simulink model "Child2"  (R2023a)
settings: Solver=FixedStepAuto  StartTime=0.0  StopTime=10.0  RelTol=1e-3
libraries: androidaudiovideolib x3, androidcommunicationlib x3, androidsensorlib x2, androiduilib x2, fuzblock x1
settings Model: Creator=srira  LastModifiedBy=srira
settings OptimizationCC: EnhancedBackFolding=on  PassReuseOutputArgsAs=Individual arguments  ZeroExternalMemoryAtStartup=off  ZeroInternalMemoryAtStartup=off  MaxStackSize=64  OptimizeBlockOrder=speed  DifferentSizesBufferReuse=on  OptimizationCustomize=off  EfficientTunableParamExpr=on
settings DebuggingCC: ParameterTunabilityLossMsg=error
settings HardwareCC: ProdBitPerPointer=32  ProdBitPerSizeT=32  ProdBitPerPtrDiffT=32  ProdLargestAtomicInteger=Long  ProdLargestAtomicFloat=Double  ProdWordSize=32  ProdHWDeviceType=ARM Compatible->ARM Cortex  UseEmbeddedCoderFeatures=off  UseSimulinkCoderFeatures=off
settings SFSimCC: MATLABDynamicMemAlloc=off
settings RTWCC: Description=Embedded Coder  SystemTargetFile=ert.tlc  HardwareBoard=Android Device  TLCOptions="-aInlineSetEventsForThisBaseRateFcn=TLC_FALSE -aSuppressMultiTaskScheduler=TLC_FALSE  -aRateBasedStepFcn=0"  TemplateMakefile=ert_default_tmf  RTWVerbose=off  Toolchain=Android SDK/NDK Tools
settings CodeAppCC: ForceParamTrailComments=on  IgnoreCustomStorageClasses=off  OperatorAnnotations=on  SimulinkDataObjDesc=on  SFDataObjDesc=on  InsertBlockDesc=on
settings ERTTargetCC: SupportNonInlinedSFcns=on

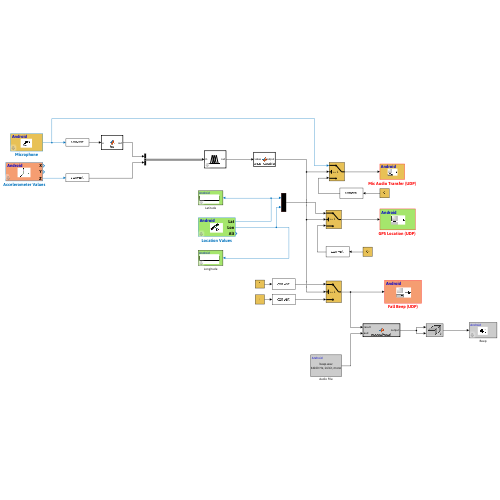
[thumbnail: Simulink's stored preview of the top-level diagram]
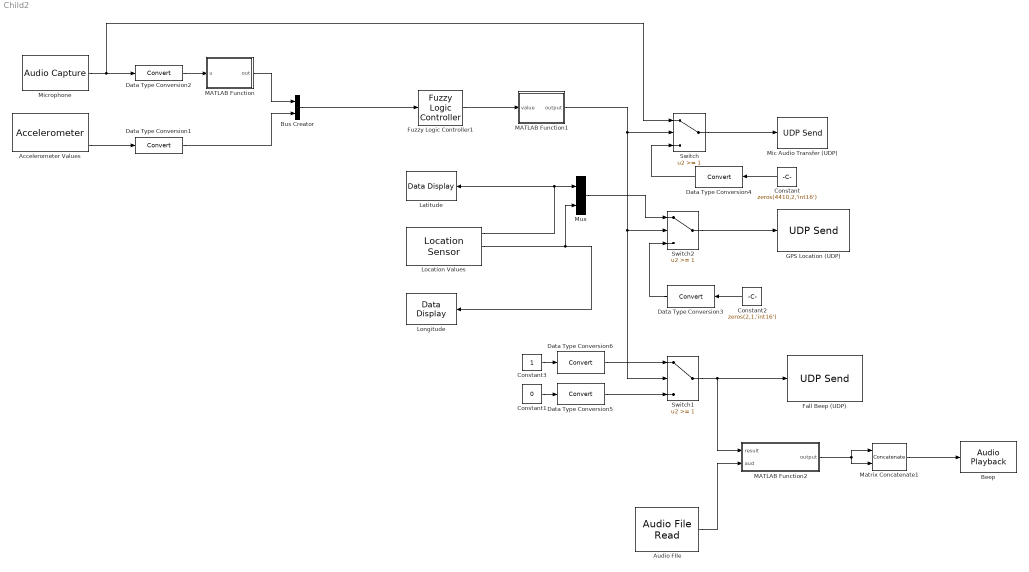
== system Child2 ==
  Accelerometer Values : androidsensorlib/Accelerometer  OutputVector=off  SampleTime=0.1  BlockPlatform=Android
  Audio FIle : androidaudiovideolib/Audio File Read  FileName=E:\IITGN\Child_Safety\beep.wav  FrameSize=4410
  Beep : androidaudiovideolib/Audio Playback  SampleFreq=44100  AudioSamplingFreq=44100  SampleTime=0.1  DeviceStr=0  QueueDuration=0  BlockPlatform=Android
  Bus Creator : BusCreator  Inputs=2
  Constant : Constant  Value=zeros(4410,2,'int16')  VectorParams1D=off
  Constant1 : Constant  Value=0  VectorParams1D=off  OutDataTypeStr=Inherit: Inherit via back propagation
  Constant2 : Constant  Value=zeros(2,1,'int16')  VectorParams1D=off  OutDataTypeStr=Inherit: Inherit via back propagation
  Constant3 : Constant  VectorParams1D=off  OutDataTypeStr=Inherit: Inherit via back propagation
  Data Type Conversion{1..6} (6 alike) : DataTypeConversion  SaturateOnIntegerOverflow=off  RndMeth=Floor
  Fall Beep (UDP) : androidcommunicationlib/UDP Send  remoteURL='10.7.59.190'  remotePort=25001  localURL='0.0.0.0'  localPortSource=Automatically determine  localPort=-1  sampletime=-1  blockPlatform=Android  separateLengthPort=0
  Fuzzy Logic Controller1 : fuzblock/Fuzzy Logic  Controller  FIS='Control_Systems.fis'  OutputSampleNumber=101  DataType=double  FuzzifiedInputs=off  RuleFiringStrengths=off  RuleOutputs=off  AggregatedOutputs=off  SimulateUsing=Interpreted execution  OutOfRangeInputValueMessage=warning  NoRuleFiredMessage=warning  EmptyOutputFuzzySetMessage=warning
  "GPS Location (UDP) " : androidcommunicationlib/UDP Send  remoteURL='10.7.59.190'  remotePort=25000  localURL='0.0.0.0'  localPortSource=Automatically determine  localPort=-1  sampletime=-1  blockPlatform=Android  separateLengthPort=0
  Latitude : androiduilib/Data Display  DataDisplayId=Child2/Latitude  Format=Float  Precision=10  SimulateUsing=Code generation  blockPlatform=Android
  Location Values : androidsensorlib/Location Sensor  OutputVector=off  SampleTime=0.1  BlockPlatform=Android
  Longitude : androiduilib/Data Display  DataDisplayId=Child2/Longitude  Format=Float  Precision=10  SimulateUsing=Code generation  blockPlatform=Android
  MATLAB Function : MATLAB Function  TreatAsAtomicUnit=on
  MATLAB Function1 : MATLAB Function  TreatAsAtomicUnit=on
  MATLAB Function2 : MATLAB Function  TreatAsAtomicUnit=on
  Matrix Concatenate1 : Concatenate  Mode=Multidimensional array  ConcatenateDimension=2
  Mic Audio Transfer (UDP) : androidcommunicationlib/UDP Send  remoteURL='10.7.59.190'  remotePort=25004  localURL='0.0.0.0'  localPortSource=Automatically determine  localPort=-1  sampletime=-1  blockPlatform=Android  separateLengthPort=0
  Microphone : androidaudiovideolib/Audio Capture  SampleFreq=44100  FrameSize=4410  SampleTime=0.1  SimulateUsing=Code generation  DeviceStr=0  QueueDuration=0  BlockPlatform=Android  AudioSamplingFreq=44100
  Mux : Mux  Inputs=2
  Switch : Switch  Threshold=1  SaturateOnIntegerOverflow=off  InputSameDT=off
  Switch1 : Switch  Threshold=1  OutDataTypeStr=Inherit: Inherit via back propagation  SaturateOnIntegerOverflow=off  InputSameDT=off
  Switch2 : Switch  Threshold=1  OutDataTypeStr=Inherit: Inherit via back propagation  SaturateOnIntegerOverflow=off  InputSameDT=off
  wires:
  Constant/1 -> Data Type Conversion4/1
  Constant2/1 -> Data Type Conversion3/1
  Mux/1 -> Switch2/1
  Microphone/1 -> Switch/1, Data Type Conversion2/1
  Fuzzy Logic Controller1/1 -> MATLAB Function1/1(value)
  Data Type Conversion1/1 -> Bus Creator/2
  MATLAB Function2/1(output) -> Matrix Concatenate1/2, Matrix Concatenate1/1
  Matrix Concatenate1/1 -> Beep/1
  Accelerometer Values/3 -> Data Type Conversion1/1
  Location Values/1 -> Latitude/1, Mux/1
  Location Values/2 -> Mux/2, Longitude/1
  Audio FIle/1 -> MATLAB Function2/2(aud)
  MATLAB Function/1(out) -> Bus Creator/1
  Switch/1 -> Mic Audio Transfer (UDP)/1
  Switch2/1 -> "GPS Location (UDP) "/1
  Data Type Conversion2/1 -> MATLAB Function/1(u)
  Bus Creator/1 -> Fuzzy Logic Controller1/1
  Data Type Conversion3/1 -> Switch2/3
  Data Type Conversion4/1 -> Switch/3
  Switch1/1 -> Fall Beep (UDP)/1, MATLAB Function2/1(result)
  Data Type Conversion5/1 -> Switch1/3
  Constant1/1 -> Data Type Conversion5/1
  Constant3/1 -> Data Type Conversion6/1
  MATLAB Function1/1(output) -> Switch1/2, Switch2/2, Switch/2
  Data Type Conversion6/1 -> Switch1/1

== matlab function Child2/MATLAB Function ==
  data: u input; out output
 function out = fcn(u)

avg_col1 = mean(abs(u(:, 1)));
avg_col2 = mean(abs(u(:, 2)));

out = max([avg_col1, avg_col2]);

== matlab function Child2/MATLAB Function2 ==
  data: result input; output output; aud input
function output = processResult(result, aud)
    if result == 1
        output = aud;
    else
        output = zeros(4410,1,'int16');
    end
end

== matlab function Child2/MATLAB Function1 ==
  data: value input; output output
function output = range_classifier(value)
  % Define ranges as cell array for readability
  ranges = {[0, 30], [30, 70], [70, 100]};
  
  % Loop through each range and check if the value falls within
  for i = 1:length(ranges)
    lower = ranges{i}(1);
    upper = ranges{i}(2);
    if (value >= lower) && (value < upper)
      output = i - 1;  % Adjust index for 0-based output (0, 1, 2)
      return;
    end
  end
  
  % If value doesn't fall within any range, return -1 (or any other value)
  output = -1;  % You can modify this value as needed (e.g., NaN)
end
